simulink model "ORGateSwitch"  (R2023a)
settings: Solver=VariableStepAuto  StartTime=0.0  StopTime=10.0  RelTol=1e-3
settings Model: Creator=aan18022  LastModifiedBy=aan18022

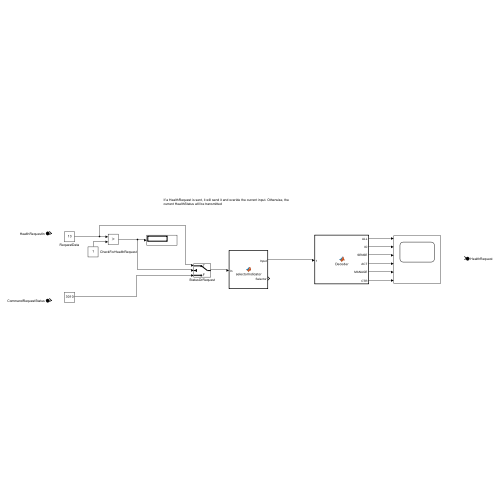
[thumbnail: Simulink's stored preview of the top-level diagram]
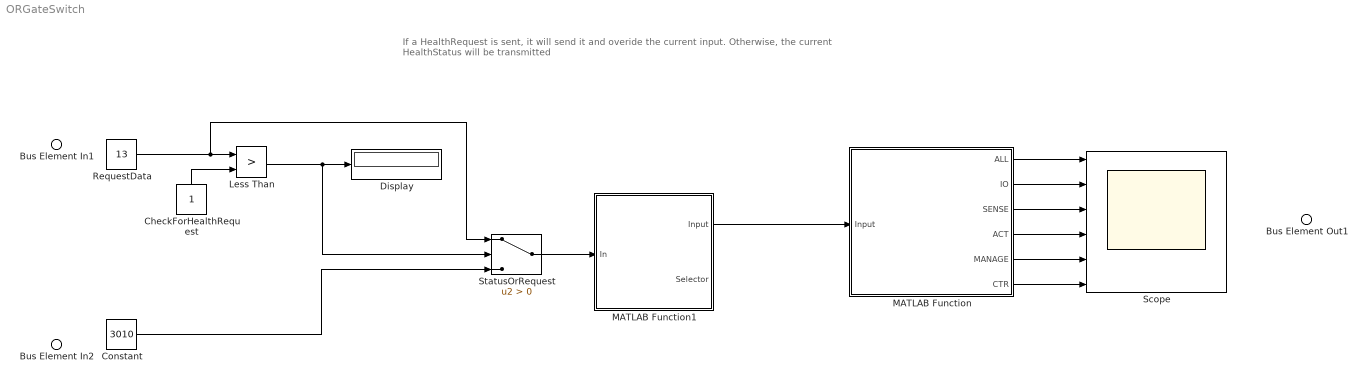
== system ORGateSwitch ==
  note: If a HealthRequest is sent, it will send it and overide the current input. Otherwise, the current HealthStatus will be transmitted
  Bus Element In1 : Inport  PortName=HealthRequestIn
  Bus Element In2 : Inport  Port=2  PortName=CommandRequestStatus
  CheckForHealthRequest : Constant
  Constant : Constant  Value=3010
  Display : Display
  Less Than : RelationalOperator  Operator=>  OutDataTypeStr=boolean  RndMeth=Simplest  InputSameDT=off
  MATLAB Function : MATLAB Function  TreatAsAtomicUnit=on
  MATLAB Function1 : MATLAB Function  TreatAsAtomicUnit=on
  RequestData : Constant  Value=13
  Scope : Scope  NumInputPorts=6
  StatusOrRequest : Switch  Criteria=u2 > Threshold  SaturateOnIntegerOverflow=off  InputSameDT=off
  Bus Element Out1 : Outport  PortName=HealthRequest
  wires:
  CheckForHealthRequest/1 -> Less Than/2
  RequestData/1 -> StatusOrRequest/1, Less Than/1
  Less Than/1 -> Display/1, StatusOrRequest/2
  MATLAB Function/3(SENSE) -> Scope/3
  MATLAB Function/2(IO) -> Scope/2
  MATLAB Function/1(ALL) -> Scope/1
  MATLAB Function/4(ACT) -> Scope/4
  MATLAB Function/5(MANAGE) -> Scope/5
  MATLAB Function/6(CTR) -> Scope/6
  Constant/1 -> StatusOrRequest/3
  StatusOrRequest/1 -> MATLAB Function1/1(In)
  MATLAB Function1/1(Input) -> MATLAB Function/1(Input)

== matlab function ORGateSwitch/MATLAB Function1 ==
  data: In input; Out output; Selector output
function [Out,Selector]= selectorIndicator(In)
result  = In -3000;
if (In < 3000)
    
    Out = In;
    Selector = 1;
else
    Out = result;
    Selector = 0;
end

== matlab function ORGateSwitch/MATLAB Function ==
  data: Input input; ALL output; IO output; SENSE output; ACT output; MANAGE output; CTR output
function [ALL,IO,SENSE,ACT,MANAGE,CTR]= Decoder(Input)

al = mod(Input,13);%All
io  = mod(Input,11);
s  = mod(Input,7);
ac = mod(Input,5);
m  = mod(Input,3);
c  = mod(Input,2);

if (al == 0)
    ALL = 1;
else
    ALL = 0;
end

if (io == 0)
    IO = 1;
else
    IO = 0;
end

if (s == 0)
    SENSE = 1;
else
    SENSE = 0;
end

if (ac == 0)
    ACT = 1;
else
    ACT = 0;    
end

if (m == 0)
    MANAGE = 1;
else
    MANAGE = 0;
end

if (c == 0)
    CTR = 1;
else
    CTR = 0;
end
